simulink model "elevatorMod"  (R2020a)
settings: Solver=VariableStepAuto  StartTime=0.0  StopTime=inf  RelTol=1e-3
PreLoadFcn:
  | slplc.api.loadDataTypes;
undefined symbols (not defined in the file): BOOL, DINT, INT, slplc
libraries: simulink x1
(part 26 of 39)

== system elevatorMod/PLCControllerSuite/__Logic/Task/Program/__Logic/OTE24/Instruction_Enable/Rung-condition is false ==
  Enable : EnablePort
  Constant : Constant  Value=0  OutDataTypeStr=BOOL
  __CoreVarWrite : Subsystem  Tag=CoreVarWriteBlock  DisableCoverage=on  TreatAsAtomicUnit=on  mask{PLCBlockType=CoreVarWrite}
      mask init:
      | slplc.callbacks.initCoreVariable(gcb, 'write');
      mask Help: web([docroot '/plccoder/ref/__corevarwrite' '.html']);
      mask DialogControl PLCBlockTitle Prompt: Core Variable Write
  wires:
  Constant/1 -> __CoreVarWrite/1(u)

== system elevatorMod/PLCControllerSuite/__Logic/Task/Program/__Logic/OTE24/Instruction_Enable/Rung-condition-in is true ==
  Enable : EnablePort
  Constant : Constant  OutDataTypeStr=BOOL
  __CoreVarWrite : Subsystem  Tag=CoreVarWriteBlock  DisableCoverage=on  TreatAsAtomicUnit=on  mask{PLCBlockType=CoreVarWrite}
      mask init:
      | slplc.callbacks.initCoreVariable(gcb, 'write');
      mask Help: web([docroot '/plccoder/ref/__corevarwrite' '.html']);
      mask DialogControl PLCBlockTitle Prompt: Core Variable Write
  wires:
  Constant/1 -> __CoreVarWrite/1(u)

== system elevatorMod/PLCControllerSuite/__Logic/Task/Program/__Logic/OTE24/RungInOverride/ForceRungInFalseRead ==
  __CoreLabelRead : Subsystem  Tag=CoreVarReadBlock  DisableCoverage=on  TreatAsAtomicUnit=on  mask{PLCBlockType=CoreLabelRead}
      mask init:
      | slplc.callbacks.initRoutineLabelRead(gcb);
      mask Help: web([docroot '/plccoder/ref/__corelabelread' '.html']);
      mask DialogControl PLCBlockTitle Prompt: Core Label Read
  Out1 : Outport  VectorParamsAs1DForOutWhenUnconnected=off
  wires:
  __CoreLabelRead/1(Out1) -> Out1/1

== system elevatorMod/PLCControllerSuite/__Logic/Task/Program/__Logic/OTE25/BlockEnableRead/__CoreLabelRead ==
  DataRead : DataStoreRead  DataStoreName=x_PLCLabel__s4_3653__Block_Enable
  Out1 : Outport  VectorParamsAs1DForOutWhenUnconnected=off
  wires:
  DataRead/1 -> Out1/1

== system elevatorMod/PLCControllerSuite/__Logic/Task/Program/__Logic/OTE25/Instruction_Enable/Initialize Function ==
  Constant : Constant  Value=0  OutDataTypeStr=BOOL
  Event Listener : EventListener  DisableCoverage=on  EventName=reset
  __CoreVarWrite : Subsystem  Tag=CoreVarWriteBlock  DisableCoverage=on  TreatAsAtomicUnit=on  mask{PLCBlockType=CoreVarWrite}
      mask init:
      | slplc.callbacks.initCoreVariable(gcb, 'write');
      mask Help: web([docroot '/plccoder/ref/__corevarwrite' '.html']);
      mask DialogControl PLCBlockTitle Prompt: Core Variable Write
  wires:
  Constant/1 -> __CoreVarWrite/1(u)

== system elevatorMod/PLCControllerSuite/__Logic/Task/Program/__Logic/OTE25/Instruction_Enable/Rung-condition is false ==
  Enable : EnablePort
  Constant : Constant  Value=0  OutDataTypeStr=BOOL
  __CoreVarWrite : Subsystem  Tag=CoreVarWriteBlock  DisableCoverage=on  TreatAsAtomicUnit=on  mask{PLCBlockType=CoreVarWrite}
      mask init:
      | slplc.callbacks.initCoreVariable(gcb, 'write');
      mask Help: web([docroot '/plccoder/ref/__corevarwrite' '.html']);
      mask DialogControl PLCBlockTitle Prompt: Core Variable Write
  wires:
  Constant/1 -> __CoreVarWrite/1(u)

== system elevatorMod/PLCControllerSuite/__Logic/Task/Program/__Logic/OTE25/Instruction_Enable/Rung-condition-in is true ==
  Enable : EnablePort
  Constant : Constant  OutDataTypeStr=BOOL
  __CoreVarWrite : Subsystem  Tag=CoreVarWriteBlock  DisableCoverage=on  TreatAsAtomicUnit=on  mask{PLCBlockType=CoreVarWrite}
      mask init:
      | slplc.callbacks.initCoreVariable(gcb, 'write');
      mask Help: web([docroot '/plccoder/ref/__corevarwrite' '.html']);
      mask DialogControl PLCBlockTitle Prompt: Core Variable Write
  wires:
  Constant/1 -> __CoreVarWrite/1(u)

== system elevatorMod/PLCControllerSuite/__Logic/Task/Program/__Logic/OTE25/RungInOverride/ForceRungInFalseRead ==
  __CoreLabelRead : Subsystem  Tag=CoreVarReadBlock  DisableCoverage=on  TreatAsAtomicUnit=on  mask{PLCBlockType=CoreLabelRead}
      mask init:
      | slplc.callbacks.initRoutineLabelRead(gcb);
      mask Help: web([docroot '/plccoder/ref/__corelabelread' '.html']);
      mask DialogControl PLCBlockTitle Prompt: Core Label Read
  Out1 : Outport  VectorParamsAs1DForOutWhenUnconnected=off
  wires:
  __CoreLabelRead/1(Out1) -> Out1/1

== system elevatorMod/PLCControllerSuite/__Logic/Task/Program/__Logic/OTE26/BlockEnableRead/__CoreLabelRead ==
  DataRead : DataStoreRead  DataStoreName=x_PLCLabel__s4_3653__Block_Enable
  Out1 : Outport  VectorParamsAs1DForOutWhenUnconnected=off
  wires:
  DataRead/1 -> Out1/1

== system elevatorMod/PLCControllerSuite/__Logic/Task/Program/__Logic/OTE26/Instruction_Enable/Initialize Function ==
  Constant : Constant  Value=0  OutDataTypeStr=BOOL
  Event Listener : EventListener  DisableCoverage=on  EventName=reset
  __CoreVarWrite : Subsystem  Tag=CoreVarWriteBlock  DisableCoverage=on  TreatAsAtomicUnit=on  mask{PLCBlockType=CoreVarWrite}
      mask init:
      | slplc.callbacks.initCoreVariable(gcb, 'write');
      mask Help: web([docroot '/plccoder/ref/__corevarwrite' '.html']);
      mask DialogControl PLCBlockTitle Prompt: Core Variable Write
  wires:
  Constant/1 -> __CoreVarWrite/1(u)

== system elevatorMod/PLCControllerSuite/__Logic/Task/Program/__Logic/OTE26/Instruction_Enable/Rung-condition is false ==
  Enable : EnablePort
  Constant : Constant  Value=0  OutDataTypeStr=BOOL
  __CoreVarWrite : Subsystem  Tag=CoreVarWriteBlock  DisableCoverage=on  TreatAsAtomicUnit=on  mask{PLCBlockType=CoreVarWrite}
      mask init:
      | slplc.callbacks.initCoreVariable(gcb, 'write');
      mask Help: web([docroot '/plccoder/ref/__corevarwrite' '.html']);
      mask DialogControl PLCBlockTitle Prompt: Core Variable Write
  wires:
  Constant/1 -> __CoreVarWrite/1(u)

== system elevatorMod/PLCControllerSuite/__Logic/Task/Program/__Logic/OTE26/Instruction_Enable/Rung-condition-in is true ==
  Enable : EnablePort
  Constant : Constant  OutDataTypeStr=BOOL
  __CoreVarWrite : Subsystem  Tag=CoreVarWriteBlock  DisableCoverage=on  TreatAsAtomicUnit=on  mask{PLCBlockType=CoreVarWrite}
      mask init:
      | slplc.callbacks.initCoreVariable(gcb, 'write');
      mask Help: web([docroot '/plccoder/ref/__corevarwrite' '.html']);
      mask DialogControl PLCBlockTitle Prompt: Core Variable Write
  wires:
  Constant/1 -> __CoreVarWrite/1(u)

== system elevatorMod/PLCControllerSuite/__Logic/Task/Program/__Logic/OTE26/RungInOverride/ForceRungInFalseRead ==
  __CoreLabelRead : Subsystem  Tag=CoreVarReadBlock  DisableCoverage=on  TreatAsAtomicUnit=on  mask{PLCBlockType=CoreLabelRead}
      mask init:
      | slplc.callbacks.initRoutineLabelRead(gcb);
      mask Help: web([docroot '/plccoder/ref/__corelabelread' '.html']);
      mask DialogControl PLCBlockTitle Prompt: Core Label Read
  Out1 : Outport  VectorParamsAs1DForOutWhenUnconnected=off
  wires:
  __CoreLabelRead/1(Out1) -> Out1/1

== system elevatorMod/PLCControllerSuite/__Logic/Task/Program/__Logic/OTE27/BlockEnableRead/__CoreLabelRead ==
  DataRead : DataStoreRead  DataStoreName=x_PLCLabel__s4_3653__Block_Enable
  Out1 : Outport  VectorParamsAs1DForOutWhenUnconnected=off
  wires:
  DataRead/1 -> Out1/1

== system elevatorMod/PLCControllerSuite/__Logic/Task/Program/__Logic/OTE27/Instruction_Enable/Initialize Function ==
  Constant : Constant  Value=0  OutDataTypeStr=BOOL
  Event Listener : EventListener  DisableCoverage=on  EventName=reset
  __CoreVarWrite : Subsystem  Tag=CoreVarWriteBlock  DisableCoverage=on  TreatAsAtomicUnit=on  mask{PLCBlockType=CoreVarWrite}
      mask init:
      | slplc.callbacks.initCoreVariable(gcb, 'write');
      mask Help: web([docroot '/plccoder/ref/__corevarwrite' '.html']);
      mask DialogControl PLCBlockTitle Prompt: Core Variable Write
  wires:
  Constant/1 -> __CoreVarWrite/1(u)

== system elevatorMod/PLCControllerSuite/__Logic/Task/Program/__Logic/OTE27/Instruction_Enable/Rung-condition is false ==
  Enable : EnablePort
  Constant : Constant  Value=0  OutDataTypeStr=BOOL
  __CoreVarWrite : Subsystem  Tag=CoreVarWriteBlock  DisableCoverage=on  TreatAsAtomicUnit=on  mask{PLCBlockType=CoreVarWrite}
      mask init:
      | slplc.callbacks.initCoreVariable(gcb, 'write');
      mask Help: web([docroot '/plccoder/ref/__corevarwrite' '.html']);
      mask DialogControl PLCBlockTitle Prompt: Core Variable Write
  wires:
  Constant/1 -> __CoreVarWrite/1(u)

== system elevatorMod/PLCControllerSuite/__Logic/Task/Program/__Logic/OTE27/Instruction_Enable/Rung-condition-in is true ==
  Enable : EnablePort
  Constant : Constant  OutDataTypeStr=BOOL
  __CoreVarWrite : Subsystem  Tag=CoreVarWriteBlock  DisableCoverage=on  TreatAsAtomicUnit=on  mask{PLCBlockType=CoreVarWrite}
      mask init:
      | slplc.callbacks.initCoreVariable(gcb, 'write');
      mask Help: web([docroot '/plccoder/ref/__corevarwrite' '.html']);
      mask DialogControl PLCBlockTitle Prompt: Core Variable Write
  wires:
  Constant/1 -> __CoreVarWrite/1(u)

== system elevatorMod/PLCControllerSuite/__Logic/Task/Program/__Logic/OTE27/RungInOverride/ForceRungInFalseRead ==
  __CoreLabelRead : Subsystem  Tag=CoreVarReadBlock  DisableCoverage=on  TreatAsAtomicUnit=on  mask{PLCBlockType=CoreLabelRead}
      mask init:
      | slplc.callbacks.initRoutineLabelRead(gcb);
      mask Help: web([docroot '/plccoder/ref/__corelabelread' '.html']);
      mask DialogControl PLCBlockTitle Prompt: Core Label Read
  Out1 : Outport  VectorParamsAs1DForOutWhenUnconnected=off
  wires:
  __CoreLabelRead/1(Out1) -> Out1/1

== system elevatorMod/PLCControllerSuite/__Logic/Task/Program/__Logic/OTE28/BlockEnableRead/__CoreLabelRead ==
  DataRead : DataStoreRead  DataStoreName=x_PLCLabel__s4_3653__Block_Enable
  Out1 : Outport  VectorParamsAs1DForOutWhenUnconnected=off
  wires:
  DataRead/1 -> Out1/1

== system elevatorMod/PLCControllerSuite/__Logic/Task/Program/__Logic/OTE28/Instruction_Enable/Initialize Function ==
  Constant : Constant  Value=0  OutDataTypeStr=BOOL
  Event Listener : EventListener  DisableCoverage=on  EventName=reset
  __CoreVarWrite : Subsystem  Tag=CoreVarWriteBlock  DisableCoverage=on  TreatAsAtomicUnit=on  mask{PLCBlockType=CoreVarWrite}
      mask init:
      | slplc.callbacks.initCoreVariable(gcb, 'write');
      mask Help: web([docroot '/plccoder/ref/__corevarwrite' '.html']);
      mask DialogControl PLCBlockTitle Prompt: Core Variable Write
  wires:
  Constant/1 -> __CoreVarWrite/1(u)

== system elevatorMod/PLCControllerSuite/__Logic/Task/Program/__Logic/OTE28/Instruction_Enable/Rung-condition is false ==
  Enable : EnablePort
  Constant : Constant  Value=0  OutDataTypeStr=BOOL
  __CoreVarWrite : Subsystem  Tag=CoreVarWriteBlock  DisableCoverage=on  TreatAsAtomicUnit=on  mask{PLCBlockType=CoreVarWrite}
      mask init:
      | slplc.callbacks.initCoreVariable(gcb, 'write');
      mask Help: web([docroot '/plccoder/ref/__corevarwrite' '.html']);
      mask DialogControl PLCBlockTitle Prompt: Core Variable Write
  wires:
  Constant/1 -> __CoreVarWrite/1(u)

== system elevatorMod/PLCControllerSuite/__Logic/Task/Program/__Logic/OTE28/Instruction_Enable/Rung-condition-in is true ==
  Enable : EnablePort
  Constant : Constant  OutDataTypeStr=BOOL
  __CoreVarWrite : Subsystem  Tag=CoreVarWriteBlock  DisableCoverage=on  TreatAsAtomicUnit=on  mask{PLCBlockType=CoreVarWrite}
      mask init:
      | slplc.callbacks.initCoreVariable(gcb, 'write');
      mask Help: web([docroot '/plccoder/ref/__corevarwrite' '.html']);
      mask DialogControl PLCBlockTitle Prompt: Core Variable Write
  wires:
  Constant/1 -> __CoreVarWrite/1(u)

== system elevatorMod/PLCControllerSuite/__Logic/Task/Program/__Logic/OTE28/RungInOverride/ForceRungInFalseRead ==
  __CoreLabelRead : Subsystem  Tag=CoreVarReadBlock  DisableCoverage=on  TreatAsAtomicUnit=on  mask{PLCBlockType=CoreLabelRead}
      mask init:
      | slplc.callbacks.initRoutineLabelRead(gcb);
      mask Help: web([docroot '/plccoder/ref/__corelabelread' '.html']);
      mask DialogControl PLCBlockTitle Prompt: Core Label Read
  Out1 : Outport  VectorParamsAs1DForOutWhenUnconnected=off
  wires:
  __CoreLabelRead/1(Out1) -> Out1/1

== system elevatorMod/PLCControllerSuite/__Logic/Task/Program/__Logic/OTE29/BlockEnableRead/__CoreLabelRead ==
  DataRead : DataStoreRead  DataStoreName=x_PLCLabel__s4_3653__Block_Enable
  Out1 : Outport  VectorParamsAs1DForOutWhenUnconnected=off
  wires:
  DataRead/1 -> Out1/1

== system elevatorMod/PLCControllerSuite/__Logic/Task/Program/__Logic/OTE29/Instruction_Enable/Initialize Function ==
  Constant : Constant  Value=0  OutDataTypeStr=BOOL
  Event Listener : EventListener  DisableCoverage=on  EventName=reset
  __CoreVarWrite : Subsystem  Tag=CoreVarWriteBlock  DisableCoverage=on  TreatAsAtomicUnit=on  mask{PLCBlockType=CoreVarWrite}
      mask init:
      | slplc.callbacks.initCoreVariable(gcb, 'write');
      mask Help: web([docroot '/plccoder/ref/__corevarwrite' '.html']);
      mask DialogControl PLCBlockTitle Prompt: Core Variable Write
  wires:
  Constant/1 -> __CoreVarWrite/1(u)

== system elevatorMod/PLCControllerSuite/__Logic/Task/Program/__Logic/OTE29/Instruction_Enable/Rung-condition is false ==
  Enable : EnablePort
  Constant : Constant  Value=0  OutDataTypeStr=BOOL
  __CoreVarWrite : Subsystem  Tag=CoreVarWriteBlock  DisableCoverage=on  TreatAsAtomicUnit=on  mask{PLCBlockType=CoreVarWrite}
      mask init:
      | slplc.callbacks.initCoreVariable(gcb, 'write');
      mask Help: web([docroot '/plccoder/ref/__corevarwrite' '.html']);
      mask DialogControl PLCBlockTitle Prompt: Core Variable Write
  wires:
  Constant/1 -> __CoreVarWrite/1(u)

== system elevatorMod/PLCControllerSuite/__Logic/Task/Program/__Logic/OTE29/Instruction_Enable/Rung-condition-in is true ==
  Enable : EnablePort
  Constant : Constant  OutDataTypeStr=BOOL
  __CoreVarWrite : Subsystem  Tag=CoreVarWriteBlock  DisableCoverage=on  TreatAsAtomicUnit=on  mask{PLCBlockType=CoreVarWrite}
      mask init:
      | slplc.callbacks.initCoreVariable(gcb, 'write');
      mask Help: web([docroot '/plccoder/ref/__corevarwrite' '.html']);
      mask DialogControl PLCBlockTitle Prompt: Core Variable Write
  wires:
  Constant/1 -> __CoreVarWrite/1(u)

== system elevatorMod/PLCControllerSuite/__Logic/Task/Program/__Logic/OTE29/RungInOverride/ForceRungInFalseRead ==
  __CoreLabelRead : Subsystem  Tag=CoreVarReadBlock  DisableCoverage=on  TreatAsAtomicUnit=on  mask{PLCBlockType=CoreLabelRead}
      mask init:
      | slplc.callbacks.initRoutineLabelRead(gcb);
      mask Help: web([docroot '/plccoder/ref/__corelabelread' '.html']);
      mask DialogControl PLCBlockTitle Prompt: Core Label Read
  Out1 : Outport  VectorParamsAs1DForOutWhenUnconnected=off
  wires:
  __CoreLabelRead/1(Out1) -> Out1/1

== system elevatorMod/PLCControllerSuite/__Logic/Task/Program/__Logic/OTE3/BlockEnableRead/__CoreLabelRead ==
  DataRead : DataStoreRead  DataStoreName=x_PLCLabel__s4_3653__Block_Enable
  Out1 : Outport  VectorParamsAs1DForOutWhenUnconnected=off
  wires:
  DataRead/1 -> Out1/1

== system elevatorMod/PLCControllerSuite/__Logic/Task/Program/__Logic/OTE3/Instruction_Enable/Initialize Function ==
  Constant : Constant  Value=0  OutDataTypeStr=BOOL
  Event Listener : EventListener  DisableCoverage=on  EventName=reset
  __CoreVarWrite : Subsystem  Tag=CoreVarWriteBlock  DisableCoverage=on  TreatAsAtomicUnit=on  mask{PLCBlockType=CoreVarWrite}
      mask init:
      | slplc.callbacks.initCoreVariable(gcb, 'write');
      mask Help: web([docroot '/plccoder/ref/__corevarwrite' '.html']);
      mask DialogControl PLCBlockTitle Prompt: Core Variable Write
  wires:
  Constant/1 -> __CoreVarWrite/1(u)

== system elevatorMod/PLCControllerSuite/__Logic/Task/Program/__Logic/OTE3/Instruction_Enable/Rung-condition is false ==
  Enable : EnablePort
  Constant : Constant  Value=0  OutDataTypeStr=BOOL
  __CoreVarWrite : Subsystem  Tag=CoreVarWriteBlock  DisableCoverage=on  TreatAsAtomicUnit=on  mask{PLCBlockType=CoreVarWrite}
      mask init:
      | slplc.callbacks.initCoreVariable(gcb, 'write');
      mask Help: web([docroot '/plccoder/ref/__corevarwrite' '.html']);
      mask DialogControl PLCBlockTitle Prompt: Core Variable Write
  wires:
  Constant/1 -> __CoreVarWrite/1(u)

== system elevatorMod/PLCControllerSuite/__Logic/Task/Program/__Logic/OTE3/Instruction_Enable/Rung-condition-in is true ==
  Enable : EnablePort
  Constant : Constant  OutDataTypeStr=BOOL
  __CoreVarWrite : Subsystem  Tag=CoreVarWriteBlock  DisableCoverage=on  TreatAsAtomicUnit=on  mask{PLCBlockType=CoreVarWrite}
      mask init:
      | slplc.callbacks.initCoreVariable(gcb, 'write');
      mask Help: web([docroot '/plccoder/ref/__corevarwrite' '.html']);
      mask DialogControl PLCBlockTitle Prompt: Core Variable Write
  wires:
  Constant/1 -> __CoreVarWrite/1(u)

== system elevatorMod/PLCControllerSuite/__Logic/Task/Program/__Logic/OTE3/RungInOverride/ForceRungInFalseRead ==
  __CoreLabelRead : Subsystem  Tag=CoreVarReadBlock  DisableCoverage=on  TreatAsAtomicUnit=on  mask{PLCBlockType=CoreLabelRead}
      mask init:
      | slplc.callbacks.initRoutineLabelRead(gcb);
      mask Help: web([docroot '/plccoder/ref/__corelabelread' '.html']);
      mask DialogControl PLCBlockTitle Prompt: Core Label Read
  Out1 : Outport  VectorParamsAs1DForOutWhenUnconnected=off
  wires:
  __CoreLabelRead/1(Out1) -> Out1/1

== system elevatorMod/PLCControllerSuite/__Logic/Task/Program/__Logic/OTE30/BlockEnableRead/__CoreLabelRead ==
  DataRead : DataStoreRead  DataStoreName=x_PLCLabel__s4_3653__Block_Enable
  Out1 : Outport  VectorParamsAs1DForOutWhenUnconnected=off
  wires:
  DataRead/1 -> Out1/1

== system elevatorMod/PLCControllerSuite/__Logic/Task/Program/__Logic/OTE30/Instruction_Enable/Initialize Function ==
  Constant : Constant  Value=0  OutDataTypeStr=BOOL
  Event Listener : EventListener  DisableCoverage=on  EventName=reset
  __CoreVarWrite : Subsystem  Tag=CoreVarWriteBlock  DisableCoverage=on  TreatAsAtomicUnit=on  mask{PLCBlockType=CoreVarWrite}
      mask init:
      | slplc.callbacks.initCoreVariable(gcb, 'write');
      mask Help: web([docroot '/plccoder/ref/__corevarwrite' '.html']);
      mask DialogControl PLCBlockTitle Prompt: Core Variable Write
  wires:
  Constant/1 -> __CoreVarWrite/1(u)

== system elevatorMod/PLCControllerSuite/__Logic/Task/Program/__Logic/OTE30/Instruction_Enable/Rung-condition is false ==
  Enable : EnablePort
  Constant : Constant  Value=0  OutDataTypeStr=BOOL
  __CoreVarWrite : Subsystem  Tag=CoreVarWriteBlock  DisableCoverage=on  TreatAsAtomicUnit=on  mask{PLCBlockType=CoreVarWrite}
      mask init:
      | slplc.callbacks.initCoreVariable(gcb, 'write');
      mask Help: web([docroot '/plccoder/ref/__corevarwrite' '.html']);
      mask DialogControl PLCBlockTitle Prompt: Core Variable Write
  wires:
  Constant/1 -> __CoreVarWrite/1(u)

== system elevatorMod/PLCControllerSuite/__Logic/Task/Program/__Logic/OTE30/Instruction_Enable/Rung-condition-in is true ==
  Enable : EnablePort
  Constant : Constant  OutDataTypeStr=BOOL
  __CoreVarWrite : Subsystem  Tag=CoreVarWriteBlock  DisableCoverage=on  TreatAsAtomicUnit=on  mask{PLCBlockType=CoreVarWrite}
      mask init:
      | slplc.callbacks.initCoreVariable(gcb, 'write');
      mask Help: web([docroot '/plccoder/ref/__corevarwrite' '.html']);
      mask DialogControl PLCBlockTitle Prompt: Core Variable Write
  wires:
  Constant/1 -> __CoreVarWrite/1(u)

== system elevatorMod/PLCControllerSuite/__Logic/Task/Program/__Logic/OTE30/RungInOverride/ForceRungInFalseRead ==
  __CoreLabelRead : Subsystem  Tag=CoreVarReadBlock  DisableCoverage=on  TreatAsAtomicUnit=on  mask{PLCBlockType=CoreLabelRead}
      mask init:
      | slplc.callbacks.initRoutineLabelRead(gcb);
      mask Help: web([docroot '/plccoder/ref/__corelabelread' '.html']);
      mask DialogControl PLCBlockTitle Prompt: Core Label Read
  Out1 : Outport  VectorParamsAs1DForOutWhenUnconnected=off
  wires:
  __CoreLabelRead/1(Out1) -> Out1/1

== system elevatorMod/PLCControllerSuite/__Logic/Task/Program/__Logic/OTE31/BlockEnableRead/__CoreLabelRead ==
  DataRead : DataStoreRead  DataStoreName=x_PLCLabel__s4_3653__Block_Enable
  Out1 : Outport  VectorParamsAs1DForOutWhenUnconnected=off
  wires:
  DataRead/1 -> Out1/1

== system elevatorMod/PLCControllerSuite/__Logic/Task/Program/__Logic/OTE31/Instruction_Enable/Initialize Function ==
  Constant : Constant  Value=0  OutDataTypeStr=BOOL
  Event Listener : EventListener  DisableCoverage=on  EventName=reset
  __CoreVarWrite : Subsystem  Tag=CoreVarWriteBlock  DisableCoverage=on  TreatAsAtomicUnit=on  mask{PLCBlockType=CoreVarWrite}
      mask init:
      | slplc.callbacks.initCoreVariable(gcb, 'write');
      mask Help: web([docroot '/plccoder/ref/__corevarwrite' '.html']);
      mask DialogControl PLCBlockTitle Prompt: Core Variable Write
  wires:
  Constant/1 -> __CoreVarWrite/1(u)

== system elevatorMod/PLCControllerSuite/__Logic/Task/Program/__Logic/OTE31/Instruction_Enable/Rung-condition is false ==
  Enable : EnablePort
  Constant : Constant  Value=0  OutDataTypeStr=BOOL
  __CoreVarWrite : Subsystem  Tag=CoreVarWriteBlock  DisableCoverage=on  TreatAsAtomicUnit=on  mask{PLCBlockType=CoreVarWrite}
      mask init:
      | slplc.callbacks.initCoreVariable(gcb, 'write');
      mask Help: web([docroot '/plccoder/ref/__corevarwrite' '.html']);
      mask DialogControl PLCBlockTitle Prompt: Core Variable Write
  wires:
  Constant/1 -> __CoreVarWrite/1(u)

== system elevatorMod/PLCControllerSuite/__Logic/Task/Program/__Logic/OTE31/Instruction_Enable/Rung-condition-in is true ==
  Enable : EnablePort
  Constant : Constant  OutDataTypeStr=BOOL
  __CoreVarWrite : Subsystem  Tag=CoreVarWriteBlock  DisableCoverage=on  TreatAsAtomicUnit=on  mask{PLCBlockType=CoreVarWrite}
      mask init:
      | slplc.callbacks.initCoreVariable(gcb, 'write');
      mask Help: web([docroot '/plccoder/ref/__corevarwrite' '.html']);
      mask DialogControl PLCBlockTitle Prompt: Core Variable Write
  wires:
  Constant/1 -> __CoreVarWrite/1(u)

== system elevatorMod/PLCControllerSuite/__Logic/Task/Program/__Logic/OTE31/RungInOverride/ForceRungInFalseRead ==
  __CoreLabelRead : Subsystem  Tag=CoreVarReadBlock  DisableCoverage=on  TreatAsAtomicUnit=on  mask{PLCBlockType=CoreLabelRead}
      mask init:
      | slplc.callbacks.initRoutineLabelRead(gcb);
      mask Help: web([docroot '/plccoder/ref/__corelabelread' '.html']);
      mask DialogControl PLCBlockTitle Prompt: Core Label Read
  Out1 : Outport  VectorParamsAs1DForOutWhenUnconnected=off
  wires:
  __CoreLabelRead/1(Out1) -> Out1/1

== system elevatorMod/PLCControllerSuite/__Logic/Task/Program/__Logic/OTE32/BlockEnableRead/__CoreLabelRead ==
  DataRead : DataStoreRead  DataStoreName=x_PLCLabel__s4_3653__Block_Enable
  Out1 : Outport  VectorParamsAs1DForOutWhenUnconnected=off
  wires:
  DataRead/1 -> Out1/1

== system elevatorMod/PLCControllerSuite/__Logic/Task/Program/__Logic/OTE32/Instruction_Enable/Initialize Function ==
  Constant : Constant  Value=0  OutDataTypeStr=BOOL
  Event Listener : EventListener  DisableCoverage=on  EventName=reset
  __CoreVarWrite : Subsystem  Tag=CoreVarWriteBlock  DisableCoverage=on  TreatAsAtomicUnit=on  mask{PLCBlockType=CoreVarWrite}
      mask init:
      | slplc.callbacks.initCoreVariable(gcb, 'write');
      mask Help: web([docroot '/plccoder/ref/__corevarwrite' '.html']);
      mask DialogControl PLCBlockTitle Prompt: Core Variable Write
  wires:
  Constant/1 -> __CoreVarWrite/1(u)

== system elevatorMod/PLCControllerSuite/__Logic/Task/Program/__Logic/OTE32/Instruction_Enable/Rung-condition is false ==
  Enable : EnablePort
  Constant : Constant  Value=0  OutDataTypeStr=BOOL
  __CoreVarWrite : Subsystem  Tag=CoreVarWriteBlock  DisableCoverage=on  TreatAsAtomicUnit=on  mask{PLCBlockType=CoreVarWrite}
      mask init:
      | slplc.callbacks.initCoreVariable(gcb, 'write');
      mask Help: web([docroot '/plccoder/ref/__corevarwrite' '.html']);
      mask DialogControl PLCBlockTitle Prompt: Core Variable Write
  wires:
  Constant/1 -> __CoreVarWrite/1(u)

== system elevatorMod/PLCControllerSuite/__Logic/Task/Program/__Logic/OTE32/Instruction_Enable/Rung-condition-in is true ==
  Enable : EnablePort
  Constant : Constant  OutDataTypeStr=BOOL
  __CoreVarWrite : Subsystem  Tag=CoreVarWriteBlock  DisableCoverage=on  TreatAsAtomicUnit=on  mask{PLCBlockType=CoreVarWrite}
      mask init:
      | slplc.callbacks.initCoreVariable(gcb, 'write');
      mask Help: web([docroot '/plccoder/ref/__corevarwrite' '.html']);
      mask DialogControl PLCBlockTitle Prompt: Core Variable Write
  wires:
  Constant/1 -> __CoreVarWrite/1(u)

== system elevatorMod/PLCControllerSuite/__Logic/Task/Program/__Logic/OTE32/RungInOverride/ForceRungInFalseRead ==
  __CoreLabelRead : Subsystem  Tag=CoreVarReadBlock  DisableCoverage=on  TreatAsAtomicUnit=on  mask{PLCBlockType=CoreLabelRead}
      mask init:
      | slplc.callbacks.initRoutineLabelRead(gcb);
      mask Help: web([docroot '/plccoder/ref/__corelabelread' '.html']);
      mask DialogControl PLCBlockTitle Prompt: Core Label Read
  Out1 : Outport  VectorParamsAs1DForOutWhenUnconnected=off
  wires:
  __CoreLabelRead/1(Out1) -> Out1/1

== system elevatorMod/PLCControllerSuite/__Logic/Task/Program/__Logic/OTE4/BlockEnableRead/__CoreLabelRead ==
  DataRead : DataStoreRead  DataStoreName=x_PLCLabel__s4_3653__Block_Enable
  Out1 : Outport  VectorParamsAs1DForOutWhenUnconnected=off
  wires:
  DataRead/1 -> Out1/1

== system elevatorMod/PLCControllerSuite/__Logic/Task/Program/__Logic/OTE4/Instruction_Enable/Initialize Function ==
  Constant : Constant  Value=0  OutDataTypeStr=BOOL
  Event Listener : EventListener  DisableCoverage=on  EventName=reset
  __CoreVarWrite : Subsystem  Tag=CoreVarWriteBlock  DisableCoverage=on  TreatAsAtomicUnit=on  mask{PLCBlockType=CoreVarWrite}
      mask init:
      | slplc.callbacks.initCoreVariable(gcb, 'write');
      mask Help: web([docroot '/plccoder/ref/__corevarwrite' '.html']);
      mask DialogControl PLCBlockTitle Prompt: Core Variable Write
  wires:
  Constant/1 -> __CoreVarWrite/1(u)

== system elevatorMod/PLCControllerSuite/__Logic/Task/Program/__Logic/OTE4/Instruction_Enable/Rung-condition is false ==
  Enable : EnablePort
  Constant : Constant  Value=0  OutDataTypeStr=BOOL
  __CoreVarWrite : Subsystem  Tag=CoreVarWriteBlock  DisableCoverage=on  TreatAsAtomicUnit=on  mask{PLCBlockType=CoreVarWrite}
      mask init:
      | slplc.callbacks.initCoreVariable(gcb, 'write');
      mask Help: web([docroot '/plccoder/ref/__corevarwrite' '.html']);
      mask DialogControl PLCBlockTitle Prompt: Core Variable Write
  wires:
  Constant/1 -> __CoreVarWrite/1(u)

== system elevatorMod/PLCControllerSuite/__Logic/Task/Program/__Logic/OTE4/Instruction_Enable/Rung-condition-in is true ==
  Enable : EnablePort
  Constant : Constant  OutDataTypeStr=BOOL
  __CoreVarWrite : Subsystem  Tag=CoreVarWriteBlock  DisableCoverage=on  TreatAsAtomicUnit=on  mask{PLCBlockType=CoreVarWrite}
      mask init:
      | slplc.callbacks.initCoreVariable(gcb, 'write');
      mask Help: web([docroot '/plccoder/ref/__corevarwrite' '.html']);
      mask DialogControl PLCBlockTitle Prompt: Core Variable Write
  wires:
  Constant/1 -> __CoreVarWrite/1(u)

== system elevatorMod/PLCControllerSuite/__Logic/Task/Program/__Logic/OTE4/RungInOverride/ForceRungInFalseRead ==
  __CoreLabelRead : Subsystem  Tag=CoreVarReadBlock  DisableCoverage=on  TreatAsAtomicUnit=on  mask{PLCBlockType=CoreLabelRead}
      mask init:
      | slplc.callbacks.initRoutineLabelRead(gcb);
      mask Help: web([docroot '/plccoder/ref/__corelabelread' '.html']);
      mask DialogControl PLCBlockTitle Prompt: Core Label Read
  Out1 : Outport  VectorParamsAs1DForOutWhenUnconnected=off
  wires:
  __CoreLabelRead/1(Out1) -> Out1/1

== system elevatorMod/PLCControllerSuite/__Logic/Task/Program/__Logic/OTE5/BlockEnableRead/__CoreLabelRead ==
  DataRead : DataStoreRead  DataStoreName=x_PLCLabel__s4_3653__Block_Enable
  Out1 : Outport  VectorParamsAs1DForOutWhenUnconnected=off
  wires:
  DataRead/1 -> Out1/1

== system elevatorMod/PLCControllerSuite/__Logic/Task/Program/__Logic/OTE5/Instruction_Enable/Initialize Function ==
  Constant : Constant  Value=0  OutDataTypeStr=BOOL
  Event Listener : EventListener  DisableCoverage=on  EventName=reset
  __CoreVarWrite : Subsystem  Tag=CoreVarWriteBlock  DisableCoverage=on  TreatAsAtomicUnit=on  mask{PLCBlockType=CoreVarWrite}
      mask init:
      | slplc.callbacks.initCoreVariable(gcb, 'write');
      mask Help: web([docroot '/plccoder/ref/__corevarwrite' '.html']);
      mask DialogControl PLCBlockTitle Prompt: Core Variable Write
  wires:
  Constant/1 -> __CoreVarWrite/1(u)

== system elevatorMod/PLCControllerSuite/__Logic/Task/Program/__Logic/OTE5/Instruction_Enable/Rung-condition is false ==
  Enable : EnablePort
  Constant : Constant  Value=0  OutDataTypeStr=BOOL
  __CoreVarWrite : Subsystem  Tag=CoreVarWriteBlock  DisableCoverage=on  TreatAsAtomicUnit=on  mask{PLCBlockType=CoreVarWrite}
      mask init:
      | slplc.callbacks.initCoreVariable(gcb, 'write');
      mask Help: web([docroot '/plccoder/ref/__corevarwrite' '.html']);
      mask DialogControl PLCBlockTitle Prompt: Core Variable Write
  wires:
  Constant/1 -> __CoreVarWrite/1(u)

== system elevatorMod/PLCControllerSuite/__Logic/Task/Program/__Logic/OTE5/Instruction_Enable/Rung-condition-in is true ==
  Enable : EnablePort
  Constant : Constant  OutDataTypeStr=BOOL
  __CoreVarWrite : Subsystem  Tag=CoreVarWriteBlock  DisableCoverage=on  TreatAsAtomicUnit=on  mask{PLCBlockType=CoreVarWrite}
      mask init:
      | slplc.callbacks.initCoreVariable(gcb, 'write');
      mask Help: web([docroot '/plccoder/ref/__corevarwrite' '.html']);
      mask DialogControl PLCBlockTitle Prompt: Core Variable Write
  wires:
  Constant/1 -> __CoreVarWrite/1(u)

== system elevatorMod/PLCControllerSuite/__Logic/Task/Program/__Logic/OTE5/RungInOverride/ForceRungInFalseRead ==
  __CoreLabelRead : Subsystem  Tag=CoreVarReadBlock  DisableCoverage=on  TreatAsAtomicUnit=on  mask{PLCBlockType=CoreLabelRead}
      mask init:
      | slplc.callbacks.initRoutineLabelRead(gcb);
      mask Help: web([docroot '/plccoder/ref/__corelabelread' '.html']);
      mask DialogControl PLCBlockTitle Prompt: Core Label Read
  Out1 : Outport  VectorParamsAs1DForOutWhenUnconnected=off
  wires:
  __CoreLabelRead/1(Out1) -> Out1/1

== system elevatorMod/PLCControllerSuite/__Logic/Task/Program/__Logic/OTE6/BlockEnableRead/__CoreLabelRead ==
  DataRead : DataStoreRead  DataStoreName=x_PLCLabel__s4_3653__Block_Enable
  Out1 : Outport  VectorParamsAs1DForOutWhenUnconnected=off
  wires:
  DataRead/1 -> Out1/1

== system elevatorMod/PLCControllerSuite/__Logic/Task/Program/__Logic/OTE6/Instruction_Enable/Initialize Function ==
  Constant : Constant  Value=0  OutDataTypeStr=BOOL
  Event Listener : EventListener  DisableCoverage=on  EventName=reset
  __CoreVarWrite : Subsystem  Tag=CoreVarWriteBlock  DisableCoverage=on  TreatAsAtomicUnit=on  mask{PLCBlockType=CoreVarWrite}
      mask init:
      | slplc.callbacks.initCoreVariable(gcb, 'write');
      mask Help: web([docroot '/plccoder/ref/__corevarwrite' '.html']);
      mask DialogControl PLCBlockTitle Prompt: Core Variable Write
  wires:
  Constant/1 -> __CoreVarWrite/1(u)

== system elevatorMod/PLCControllerSuite/__Logic/Task/Program/__Logic/OTE6/Instruction_Enable/Rung-condition is false ==
  Enable : EnablePort
  Constant : Constant  Value=0  OutDataTypeStr=BOOL
  __CoreVarWrite : Subsystem  Tag=CoreVarWriteBlock  DisableCoverage=on  TreatAsAtomicUnit=on  mask{PLCBlockType=CoreVarWrite}
      mask init:
      | slplc.callbacks.initCoreVariable(gcb, 'write');
      mask Help: web([docroot '/plccoder/ref/__corevarwrite' '.html']);
      mask DialogControl PLCBlockTitle Prompt: Core Variable Write
  wires:
  Constant/1 -> __CoreVarWrite/1(u)

== system elevatorMod/PLCControllerSuite/__Logic/Task/Program/__Logic/OTE6/Instruction_Enable/Rung-condition-in is true ==
  Enable : EnablePort
  Constant : Constant  OutDataTypeStr=BOOL
  __CoreVarWrite : Subsystem  Tag=CoreVarWriteBlock  DisableCoverage=on  TreatAsAtomicUnit=on  mask{PLCBlockType=CoreVarWrite}
      mask init:
      | slplc.callbacks.initCoreVariable(gcb, 'write');
      mask Help: web([docroot '/plccoder/ref/__corevarwrite' '.html']);
      mask DialogControl PLCBlockTitle Prompt: Core Variable Write
  wires:
  Constant/1 -> __CoreVarWrite/1(u)

== system elevatorMod/PLCControllerSuite/__Logic/Task/Program/__Logic/OTE6/RungInOverride/ForceRungInFalseRead ==
  __CoreLabelRead : Subsystem  Tag=CoreVarReadBlock  DisableCoverage=on  TreatAsAtomicUnit=on  mask{PLCBlockType=CoreLabelRead}
      mask init:
      | slplc.callbacks.initRoutineLabelRead(gcb);
      mask Help: web([docroot '/plccoder/ref/__corelabelread' '.html']);
      mask DialogControl PLCBlockTitle Prompt: Core Label Read
  Out1 : Outport  VectorParamsAs1DForOutWhenUnconnected=off
  wires:
  __CoreLabelRead/1(Out1) -> Out1/1

== system elevatorMod/PLCControllerSuite/__Logic/Task/Program/__Logic/OTE7/BlockEnableRead/__CoreLabelRead ==
  DataRead : DataStoreRead  DataStoreName=x_PLCLabel__s4_3653__Block_Enable
  Out1 : Outport  VectorParamsAs1DForOutWhenUnconnected=off
  wires:
  DataRead/1 -> Out1/1

== system elevatorMod/PLCControllerSuite/__Logic/Task/Program/__Logic/OTE7/Instruction_Enable/Initialize Function ==
  Constant : Constant  Value=0  OutDataTypeStr=BOOL
  Event Listener : EventListener  DisableCoverage=on  EventName=reset
  __CoreVarWrite : Subsystem  Tag=CoreVarWriteBlock  DisableCoverage=on  TreatAsAtomicUnit=on  mask{PLCBlockType=CoreVarWrite}
      mask init:
      | slplc.callbacks.initCoreVariable(gcb, 'write');
      mask Help: web([docroot '/plccoder/ref/__corevarwrite' '.html']);
      mask DialogControl PLCBlockTitle Prompt: Core Variable Write
  wires:
  Constant/1 -> __CoreVarWrite/1(u)

== system elevatorMod/PLCControllerSuite/__Logic/Task/Program/__Logic/OTE7/Instruction_Enable/Rung-condition is false ==
  Enable : EnablePort
  Constant : Constant  Value=0  OutDataTypeStr=BOOL
  __CoreVarWrite : Subsystem  Tag=CoreVarWriteBlock  DisableCoverage=on  TreatAsAtomicUnit=on  mask{PLCBlockType=CoreVarWrite}
      mask init:
      | slplc.callbacks.initCoreVariable(gcb, 'write');
      mask Help: web([docroot '/plccoder/ref/__corevarwrite' '.html']);
      mask DialogControl PLCBlockTitle Prompt: Core Variable Write
  wires:
  Constant/1 -> __CoreVarWrite/1(u)

== system elevatorMod/PLCControllerSuite/__Logic/Task/Program/__Logic/OTE7/Instruction_Enable/Rung-condition-in is true ==
  Enable : EnablePort
  Constant : Constant  OutDataTypeStr=BOOL
  __CoreVarWrite : Subsystem  Tag=CoreVarWriteBlock  DisableCoverage=on  TreatAsAtomicUnit=on  mask{PLCBlockType=CoreVarWrite}
      mask init:
      | slplc.callbacks.initCoreVariable(gcb, 'write');
      mask Help: web([docroot '/plccoder/ref/__corevarwrite' '.html']);
      mask DialogControl PLCBlockTitle Prompt: Core Variable Write
  wires:
  Constant/1 -> __CoreVarWrite/1(u)

== system elevatorMod/PLCControllerSuite/__Logic/Task/Program/__Logic/OTE7/RungInOverride/ForceRungInFalseRead ==
  __CoreLabelRead : Subsystem  Tag=CoreVarReadBlock  DisableCoverage=on  TreatAsAtomicUnit=on  mask{PLCBlockType=CoreLabelRead}
      mask init:
      | slplc.callbacks.initRoutineLabelRead(gcb);
      mask Help: web([docroot '/plccoder/ref/__corelabelread' '.html']);
      mask DialogControl PLCBlockTitle Prompt: Core Label Read
  Out1 : Outport  VectorParamsAs1DForOutWhenUnconnected=off
  wires:
  __CoreLabelRead/1(Out1) -> Out1/1

== system elevatorMod/PLCControllerSuite/__Logic/Task/Program/__Logic/OTE8/BlockEnableRead/__CoreLabelRead ==
  DataRead : DataStoreRead  DataStoreName=x_PLCLabel__s4_3653__Block_Enable
  Out1 : Outport  VectorParamsAs1DForOutWhenUnconnected=off
  wires:
  DataRead/1 -> Out1/1

== system elevatorMod/PLCControllerSuite/__Logic/Task/Program/__Logic/OTE8/Instruction_Enable/Initialize Function ==
  Constant : Constant  Value=0  OutDataTypeStr=BOOL
  Event Listener : EventListener  DisableCoverage=on  EventName=reset
  __CoreVarWrite : Subsystem  Tag=CoreVarWriteBlock  DisableCoverage=on  TreatAsAtomicUnit=on  mask{PLCBlockType=CoreVarWrite}
      mask init:
      | slplc.callbacks.initCoreVariable(gcb, 'write');
      mask Help: web([docroot '/plccoder/ref/__corevarwrite' '.html']);
      mask DialogControl PLCBlockTitle Prompt: Core Variable Write
  wires:
  Constant/1 -> __CoreVarWrite/1(u)

== system elevatorMod/PLCControllerSuite/__Logic/Task/Program/__Logic/OTE8/Instruction_Enable/Rung-condition is false ==
  Enable : EnablePort
  Constant : Constant  Value=0  OutDataTypeStr=BOOL
  __CoreVarWrite : Subsystem  Tag=CoreVarWriteBlock  DisableCoverage=on  TreatAsAtomicUnit=on  mask{PLCBlockType=CoreVarWrite}
      mask init:
      | slplc.callbacks.initCoreVariable(gcb, 'write');
      mask Help: web([docroot '/plccoder/ref/__corevarwrite' '.html']);
      mask DialogControl PLCBlockTitle Prompt: Core Variable Write
  wires:
  Constant/1 -> __CoreVarWrite/1(u)

== system elevatorMod/PLCControllerSuite/__Logic/Task/Program/__Logic/OTE8/Instruction_Enable/Rung-condition-in is true ==
  Enable : EnablePort
  Constant : Constant  OutDataTypeStr=BOOL
  __CoreVarWrite : Subsystem  Tag=CoreVarWriteBlock  DisableCoverage=on  TreatAsAtomicUnit=on  mask{PLCBlockType=CoreVarWrite}
      mask init:
      | slplc.callbacks.initCoreVariable(gcb, 'write');
      mask Help: web([docroot '/plccoder/ref/__corevarwrite' '.html']);
      mask DialogControl PLCBlockTitle Prompt: Core Variable Write
  wires:
  Constant/1 -> __CoreVarWrite/1(u)

== system elevatorMod/PLCControllerSuite/__Logic/Task/Program/__Logic/OTE8/RungInOverride/ForceRungInFalseRead ==
  __CoreLabelRead : Subsystem  Tag=CoreVarReadBlock  DisableCoverage=on  TreatAsAtomicUnit=on  mask{PLCBlockType=CoreLabelRead}
      mask init:
      | slplc.callbacks.initRoutineLabelRead(gcb);
      mask Help: web([docroot '/plccoder/ref/__corelabelread' '.html']);
      mask DialogControl PLCBlockTitle Prompt: Core Label Read
  Out1 : Outport  VectorParamsAs1DForOutWhenUnconnected=off
  wires:
  __CoreLabelRead/1(Out1) -> Out1/1

== system elevatorMod/PLCControllerSuite/__Logic/Task/Program/__Logic/OTE9/BlockEnableRead/__CoreLabelRead ==
  DataRead : DataStoreRead  DataStoreName=x_PLCLabel__s4_3653__Block_Enable
  Out1 : Outport  VectorParamsAs1DForOutWhenUnconnected=off
  wires:
  DataRead/1 -> Out1/1

== system elevatorMod/PLCControllerSuite/__Logic/Task/Program/__Logic/OTE9/Instruction_Enable/Initialize Function ==
  Constant : Constant  Value=0  OutDataTypeStr=BOOL
  Event Listener : EventListener  DisableCoverage=on  EventName=reset
  __CoreVarWrite : Subsystem  Tag=CoreVarWriteBlock  DisableCoverage=on  TreatAsAtomicUnit=on  mask{PLCBlockType=CoreVarWrite}
      mask init:
      | slplc.callbacks.initCoreVariable(gcb, 'write');
      mask Help: web([docroot '/plccoder/ref/__corevarwrite' '.html']);
      mask DialogControl PLCBlockTitle Prompt: Core Variable Write
  wires:
  Constant/1 -> __CoreVarWrite/1(u)

== system elevatorMod/PLCControllerSuite/__Logic/Task/Program/__Logic/OTE9/Instruction_Enable/Rung-condition is false ==
  Enable : EnablePort
  Constant : Constant  Value=0  OutDataTypeStr=BOOL
  __CoreVarWrite : Subsystem  Tag=CoreVarWriteBlock  DisableCoverage=on  TreatAsAtomicUnit=on  mask{PLCBlockType=CoreVarWrite}
      mask init:
      | slplc.callbacks.initCoreVariable(gcb, 'write');
      mask Help: web([docroot '/plccoder/ref/__corevarwrite' '.html']);
      mask DialogControl PLCBlockTitle Prompt: Core Variable Write
  wires:
  Constant/1 -> __CoreVarWrite/1(u)

== system elevatorMod/PLCControllerSuite/__Logic/Task/Program/__Logic/OTE9/Instruction_Enable/Rung-condition-in is true ==
  Enable : EnablePort
  Constant : Constant  OutDataTypeStr=BOOL
  __CoreVarWrite : Subsystem  Tag=CoreVarWriteBlock  DisableCoverage=on  TreatAsAtomicUnit=on  mask{PLCBlockType=CoreVarWrite}
      mask init:
      | slplc.callbacks.initCoreVariable(gcb, 'write');
      mask Help: web([docroot '/plccoder/ref/__corevarwrite' '.html']);
      mask DialogControl PLCBlockTitle Prompt: Core Variable Write
  wires:
  Constant/1 -> __CoreVarWrite/1(u)

== system elevatorMod/PLCControllerSuite/__Logic/Task/Program/__Logic/OTE9/RungInOverride/ForceRungInFalseRead ==
  __CoreLabelRead : Subsystem  Tag=CoreVarReadBlock  DisableCoverage=on  TreatAsAtomicUnit=on  mask{PLCBlockType=CoreLabelRead}
      mask init:
      | slplc.callbacks.initRoutineLabelRead(gcb);
      mask Help: web([docroot '/plccoder/ref/__corelabelread' '.html']);
      mask DialogControl PLCBlockTitle Prompt: Core Label Read
  Out1 : Outport  VectorParamsAs1DForOutWhenUnconnected=off
  wires:
  __CoreLabelRead/1(Out1) -> Out1/1

== system elevatorMod/PLCControllerSuite/__Logic/Task/Program/__Logic/SUB/BlockEnableRead/__CoreLabelRead ==
  DataRead : DataStoreRead  DataStoreName=x_PLCLabel__s4_3653__Block_Enable
  Out1 : Outport  VectorParamsAs1DForOutWhenUnconnected=off
  wires:
  DataRead/1 -> Out1/1

== system elevatorMod/PLCControllerSuite/__Logic/Task/Program/__Logic/SUB/RungInOverride/ForceRungInFalseRead ==
  __CoreLabelRead : Subsystem  Tag=CoreVarReadBlock  DisableCoverage=on  TreatAsAtomicUnit=on  mask{PLCBlockType=CoreLabelRead}
      mask init:
      | slplc.callbacks.initRoutineLabelRead(gcb);
      mask Help: web([docroot '/plccoder/ref/__corelabelread' '.html']);
      mask DialogControl PLCBlockTitle Prompt: Core Label Read
  Out1 : Outport  VectorParamsAs1DForOutWhenUnconnected=off
  wires:
  __CoreLabelRead/1(Out1) -> Out1/1

== system elevatorMod/PLCControllerSuite/__Logic/Task/Program/__Logic/SUB/RungOutOverride/BlockEnableRead ==
  __CoreLabelRead : Subsystem  Tag=CoreVarReadBlock  DisableCoverage=on  TreatAsAtomicUnit=on  mask{PLCBlockType=CoreLabelRead}
      mask init:
      | slplc.callbacks.initRoutineLabelRead(gcb);
      mask Help: web([docroot '/plccoder/ref/__corelabelread' '.html']);
      mask DialogControl PLCBlockTitle Prompt: Core Label Read
  Out1 : Outport  VectorParamsAs1DForOutWhenUnconnected=off
  wires:
  __CoreLabelRead/1(Out1) -> Out1/1

== system elevatorMod/PLCControllerSuite/__Logic/Task/Program/__Logic/SUB/RungOutOverride/VariableWriteEnableWrite ==
  In1 : Inport
  __CoreLabelWrite : Subsystem  Tag=CoreVarWriteBlock  DisableCoverage=on  TreatAsAtomicUnit=on  mask{PLCBlockType=CoreLabelWrite}
      mask init:
      | slplc.callbacks.initRoutineLabelWrite(gcb);
      mask Help: web([docroot '/plccoder/ref/__corelabelwrite' '.html']);
      mask DialogControl PLCBlockTitle Prompt: Core Label Write
  wires:
  In1/1 -> __CoreLabelWrite/1(In1)

== system elevatorMod/PLCControllerSuite/__Logic/Task/Program/__Logic/TON/BlockEnableRead/__CoreLabelRead ==
  DataRead : DataStoreRead  DataStoreName=x_PLCLabel__s4_3653__Block_Enable
  Out1 : Outport  VectorParamsAs1DForOutWhenUnconnected=off
  wires:
  DataRead/1 -> Out1/1

== system elevatorMod/PLCControllerSuite/__Logic/Task/Program/__Logic/TON/Instruction_Enable/Initialize Function ==
  Constant : Constant  Value=0  OutDataTypeStr=BOOL
  Constant1 : Constant  Value=0  OutDataTypeStr=DINT
  Event Listener : EventListener  DisableCoverage=on  EventName=reset
  VarWrite : Subsystem  DisableCoverage=on  TreatAsAtomicUnit=on  mask{PLCOperandTag=ACC, PLCOperandExpression=xxx_PLC_VAR_T.ACC, PLCBlockType=VarWrite, PLCPOUType=VarWrite}
      mask prompts: PLCOperandTag "Operand Tag:"
      mask init:
      | slplc.callbacks.initInstruction(gcb);
      mask Help: web([docroot '/plccoder/ref/varwrite' '.html']);
      mask DialogControl PLCBlockTitle Prompt: Variable Write
      mask Display: disp(get_param(gcb, 'PLCOperandTag'));
  VarWrite1 : Subsystem  DisableCoverage=on  TreatAsAtomicUnit=on  mask{PLCOperandTag=EN, PLCOperandExpression=xxx_PLC_VAR_T.EN, PLCBlockType=VarWrite, PLCPOUType=VarWrite}
      mask prompts: PLCOperandTag "Operand Tag:"
      mask init:
      | slplc.callbacks.initInstruction(gcb);
      mask Help: web([docroot '/plccoder/ref/varwrite' '.html']);
      mask DialogControl PLCBlockTitle Prompt: Variable Write
      mask Display: disp(get_param(gcb, 'PLCOperandTag'));
  VarWrite2 : Subsystem  DisableCoverage=on  TreatAsAtomicUnit=on  mask{PLCOperandTag=TT, PLCOperandExpression=xxx_PLC_VAR_T.TT, PLCBlockType=VarWrite, PLCPOUType=VarWrite}
      mask prompts: PLCOperandTag "Operand Tag:"
      mask init:
      | slplc.callbacks.initInstruction(gcb);
      mask Help: web([docroot '/plccoder/ref/varwrite' '.html']);
      mask DialogControl PLCBlockTitle Prompt: Variable Write
      mask Display: disp(get_param(gcb, 'PLCOperandTag'));
  VarWrite3 : Subsystem  DisableCoverage=on  TreatAsAtomicUnit=on  mask{PLCOperandTag=DN, PLCOperandExpression=xxx_PLC_VAR_T.DN, PLCBlockType=VarWrite, PLCPOUType=VarWrite}
      mask prompts: PLCOperandTag "Operand Tag:"
      mask init:
      | slplc.callbacks.initInstruction(gcb);
      mask Help: web([docroot '/plccoder/ref/varwrite' '.html']);
      mask DialogControl PLCBlockTitle Prompt: Variable Write
      mask Display: disp(get_param(gcb, 'PLCOperandTag'));
  wires:
  Constant/1 -> VarWrite1/1(In1), VarWrite2/1(In1), VarWrite3/1(In1)
  Constant1/1 -> VarWrite/1(In1)

== system elevatorMod/PLCControllerSuite/__Logic/Task/Program/__Logic/TON/Instruction_Enable/__CoreVarRead ==
  DataRead : DataStoreRead  DataStoreName=xxx_PLC_VAR_T
  y : Outport  VectorParamsAs1DForOutWhenUnconnected=off
  wires:
  DataRead/1 -> y/1

== system elevatorMod/PLCControllerSuite/__Logic/Task/Program/__Logic/TON/Instruction_Enable/__CoreVarWrite ==
  u : Inport
  DataWrite : DataStoreWrite  DataStoreName=xxx_PLC_VAR_T
  wires:
  u/1 -> DataWrite/1

== system elevatorMod/PLCControllerSuite/__Logic/Task/Program/__Logic/TON/RungInOverride/ForceRungInFalseRead ==
  __CoreLabelRead : Subsystem  Tag=CoreVarReadBlock  DisableCoverage=on  TreatAsAtomicUnit=on  mask{PLCBlockType=CoreLabelRead}
      mask init:
      | slplc.callbacks.initRoutineLabelRead(gcb);
      mask Help: web([docroot '/plccoder/ref/__corelabelread' '.html']);
      mask DialogControl PLCBlockTitle Prompt: Core Label Read
  Out1 : Outport  VectorParamsAs1DForOutWhenUnconnected=off
  wires:
  __CoreLabelRead/1(Out1) -> Out1/1

== system elevatorMod/PLCControllerSuite/__Logic/Task/Program/__Logic/Variable Write1/VariableWriteEnableRead/__CoreLabelRead ==
  DataRead : DataStoreRead  DataStoreName=x_PLCLabel__s4_3653__Variable_Write_Enable
  Out1 : Outport  VectorParamsAs1DForOutWhenUnconnected=off
  wires:
  DataRead/1 -> Out1/1

== system elevatorMod/PLCControllerSuite/__Logic/Task/Program/__Logic/Variable Write1/__Enable/__CoreVarWrite ==
  u : Inport
  DataWrite : DataStoreWrite  DataStoreName=xxx_PLC_VAR_Current_floor
  wires:
  u/1 -> DataWrite/1

== system elevatorMod/PLCControllerSuite/__Logic/Task/Program/__Logic/Variable Write2/VariableWriteEnableRead/__CoreLabelRead ==
  DataRead : DataStoreRead  DataStoreName=x_PLCLabel__s4_3653__Variable_Write_Enable
  Out1 : Outport  VectorParamsAs1DForOutWhenUnconnected=off
  wires:
  DataRead/1 -> Out1/1

== system elevatorMod/PLCControllerSuite/__Logic/Task/Program/__Logic/Variable Write2/__Enable/__CoreVarWrite ==
  u : Inport
  DataWrite : DataStoreWrite  DataStoreName=xxx_PLC_VAR_Current_floor
  wires:
  u/1 -> DataWrite/1

== system elevatorMod/PLCControllerSuite/__Logic/Task/Program/__Logic/Variable Write3/VariableWriteEnableRead/__CoreLabelRead ==
  DataRead : DataStoreRead  DataStoreName=x_PLCLabel__s4_3653__Variable_Write_Enable
  Out1 : Outport  VectorParamsAs1DForOutWhenUnconnected=off
  wires:
  DataRead/1 -> Out1/1

== system elevatorMod/PLCControllerSuite/__Logic/Task/Program/__Logic/Variable Write3/__Enable/__CoreVarWrite ==
  u : Inport
  DataWrite : DataStoreWrite  DataStoreName=xxx_PLC_VAR_Current_floor
  wires:
  u/1 -> DataWrite/1

== system elevatorMod/PLCControllerSuite/__Logic/Task/Program/__Logic/Variable Write4/VariableWriteEnableRead/__CoreLabelRead ==
  DataRead : DataStoreRead  DataStoreName=x_PLCLabel__s4_3653__Variable_Write_Enable
  Out1 : Outport  VectorParamsAs1DForOutWhenUnconnected=off
  wires:
  DataRead/1 -> Out1/1

== system elevatorMod/PLCControllerSuite/__Logic/Task/Program/__Logic/Variable Write4/__Enable/__CoreVarWrite ==
  u : Inport
  DataWrite : DataStoreWrite  DataStoreName=xxx_PLC_VAR_VARVEL
  wires:
  u/1 -> DataWrite/1

== system elevatorMod/PLCControllerSuite/__Logic/Task/Program/__Logic/Variable Write5/VariableWriteEnableRead/__CoreLabelRead ==
  DataRead : DataStoreRead  DataStoreName=x_PLCLabel__s4_3653__Variable_Write_Enable
  Out1 : Outport  VectorParamsAs1DForOutWhenUnconnected=off
  wires:
  DataRead/1 -> Out1/1

== system elevatorMod/PLCControllerSuite/__Logic/Task/Program/__Logic/Variable Write5/__Enable/__CoreVarWrite ==
  u : Inport
  DataWrite : DataStoreWrite  DataStoreName=xxx_PLC_VAR_VARVEL
  wires:
  u/1 -> DataWrite/1

== system elevatorMod/PLCControllerSuite/__Logic/Task/Program/__Logic/Variable Write6/VariableWriteEnableRead/__CoreLabelRead ==
  DataRead : DataStoreRead  DataStoreName=x_PLCLabel__s4_3653__Variable_Write_Enable
  Out1 : Outport  VectorParamsAs1DForOutWhenUnconnected=off
  wires:
  DataRead/1 -> Out1/1

== system elevatorMod/PLCControllerSuite/__Logic/Task/Program/__Logic/Variable Write6/__Enable/__CoreVarWrite ==
  u : Inport
  DataWrite : DataStoreWrite  DataStoreName=xxx_PLC_VAR_VARVEL
  wires:
  u/1 -> DataWrite/1
